simulink model "RealEstado2"  (R2023b)
settings: Solver=VariableStepAuto  StartTime=0.0  StopTime=10.0  RelTol=1e-3
settings Model: Creator=User  LastModifiedBy=User

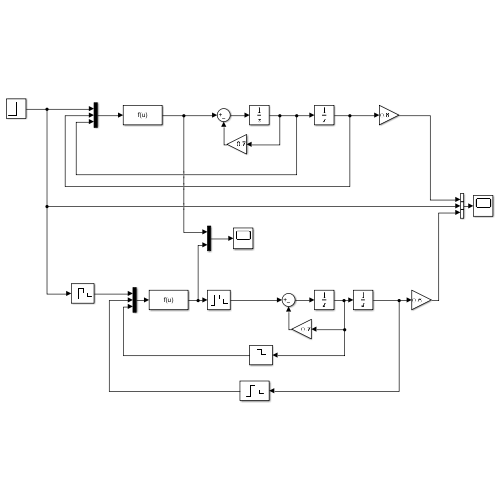
[thumbnail: Simulink's stored preview of the top-level diagram]
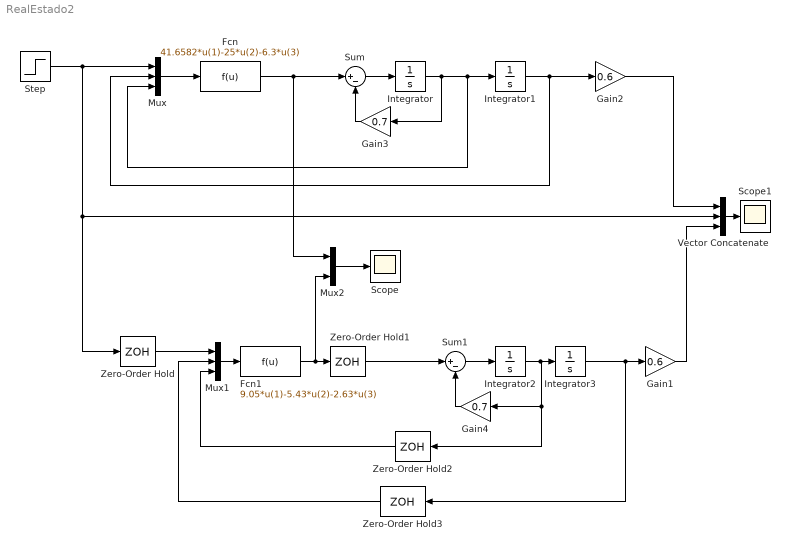
== system RealEstado2 ==
  Fcn : Fcn  Expr=41.6582*u(1)-25*u(2)-6.3*u(3)
  Fcn1 : Fcn  Expr=9.05*u(1)-5.43*u(2)-2.63*u(3)
  Gain1 : Gain  Gain=0.6
  Gain2 : Gain  Gain=0.6
  Gain3 : Gain  Gain=0.7
  Gain4 : Gain  Gain=0.7
  Integrator{,1..3} (4 alike) : Integrator
  Mux : Mux  Inputs=3
  Mux1 : Mux  Inputs=3
  Mux2 : Mux  Inputs=2
  Scope : Scope
  Scope1 : Scope
  Step : Step  SampleTime=0
  Sum : Sum  Inputs=|+-
  Sum1 : Sum  Inputs=|+-
  Vector Concatenate : Concatenate  NumInputs=3
  Zero-Order Hold{,1..3} (4 alike) : ZeroOrderHold  SampleTime=0.05
  wires:
  Mux/1 -> Fcn/1
  Vector Concatenate/1 -> Scope1/1
  Step/1 -> Vector Concatenate/2, Zero-Order Hold/1, Mux/1
  Mux1/1 -> Fcn1/1
  Zero-Order Hold/1 -> Mux1/1
  Fcn1/1 -> Mux2/2, Zero-Order Hold1/1
  Zero-Order Hold2/1 -> Mux1/3
  Zero-Order Hold3/1 -> Mux1/2
  Fcn/1 -> Mux2/1, Sum/1
  Sum/1 -> Integrator/1
  Gain3/1 -> Sum/2
  Sum1/1 -> Integrator2/1
  Zero-Order Hold1/1 -> Sum1/1
  Gain4/1 -> Sum1/2
  Integrator2/1 -> Zero-Order Hold2/1, Gain4/1, Integrator3/1
  Integrator3/1 -> Gain1/1, Zero-Order Hold3/1
  Integrator1/1 -> Gain2/1, Mux/2
  Integrator/1 -> Gain3/1, Mux/3, Integrator1/1
  Gain2/1 -> Vector Concatenate/1
  Gain1/1 -> Vector Concatenate/3
  Mux2/1 -> Scope/1
